simulink model "Subject1"  (R2022b)
settings: Solver=VariableStepAuto  StartTime=0.0  StopTime=30  RelTol=1e-3
settings Model: Creator=ParkJunHo  LastModifiedBy=ParkJunHo

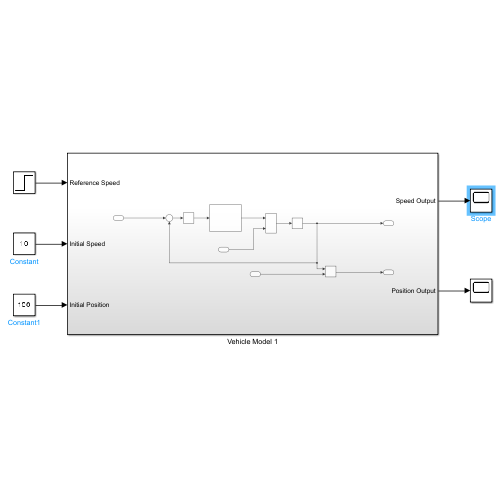
[thumbnail: Simulink's stored preview of the top-level diagram]
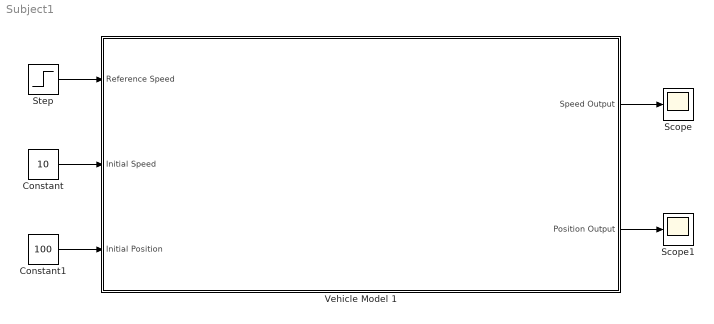
== system Subject1 ==
  Constant : Constant  Value=10
  Constant1 : Constant  Value=100
  Scope : Scope
  Scope1 : Scope
  Step : Step  Time=0  Before=20  After=20  SampleTime=0
  Vehicle Model 1 : Subsystem
  wires:
  Vehicle Model 1/1(Speed Output) -> Scope/1
  Vehicle Model 1/2(Position Output) -> Scope1/1
  Step/1 -> Vehicle Model 1/1(Reference Speed)
  Constant/1 -> Vehicle Model 1/2(Initial Speed)
  Constant1/1 -> Vehicle Model 1/3(Initial Position)

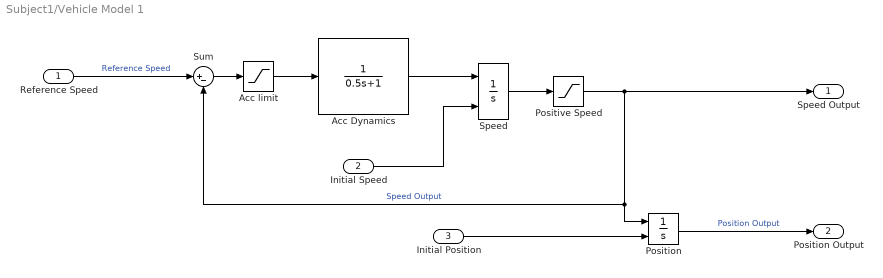
== system Subject1/Vehicle Model 1 ==
  Reference Speed : Inport
  Initial Speed : Inport  Port=2
  Initial Position : Inport  Port=3
  Acc Dynamics : TransferFcn  Denominator=[0.5 1]
  Acc limit : Saturate  UpperLimit=2  LowerLimit=-3
  Position : Integrator  InitialConditionSource=external
  Positive Speed : Saturate  UpperLimit=inf  LowerLimit=0
  Speed : Integrator  InitialConditionSource=external
  Sum : Sum  Inputs=|+-
  Speed Output : Outport
  Position Output : Outport  Port=2
  wires:
  Positive Speed/1 -> Speed Output/1, Position/1, Sum/2  "Speed Output"
  Sum/1 -> Acc limit/1
  Reference Speed/1 -> Sum/1  "Reference Speed"
  Acc limit/1 -> Acc Dynamics/1
  Initial Position/1 -> Position/2
  Acc Dynamics/1 -> Speed/1
  Speed/1 -> Positive Speed/1
  Position/1 -> Position Output/1  "Position Output"
  Initial Speed/1 -> Speed/2
